simulink model "Complete_Sensorless_FOC_EKF_simulink_model"  (R2026a)
settings: Solver=ode23s  StopTime=inf  FixedStep=5e-5  MaxStep=1e-2
model workspace (MAT data in the model file):
  SL_ROS_VariableLengthArrays_MaxSizes.CommonInfo.ArrayTruncateAction = 'EmitWarning'
  SL_ROS_VariableLengthArrays_MaxSizes.MsgTypeMap = containers.Map
  SL_ROS_VariableLengthArrays_MaxSizes.MsgTypeMap.serialization.keys = {'std_msgs/Float64MultiArray'}
  SL_ROS_VariableLengthArrays_MaxSizes.MsgTypeMap.serialization.values{1}.PropertyName = 'data'
  SL_ROS_VariableLengthArrays_MaxSizes.MsgTypeMap.serialization.values{1}.DataType = 'double'
  SL_ROS_VariableLengthArrays_MaxSizes.MsgTypeMap.serialization.values{1}.MaxLength = 6
  SL_ROS_VariableLengthArrays_MaxSizes.MsgTypeMap.serialization.uniformity = 0
  SL_ROS_VariableLengthArrays_MaxSizes.MsgTypeMap.serialization.keyType = 'char'
  SL_ROS_VariableLengthArrays_MaxSizes.MsgTypeMap.serialization.valueType = 'any'
values from neighbouring files (symbols this model uses):
  id_ref = 0    [motor_params.m]
  J = 0.001    [motor_params.m]
  Kp_id = 37.7    [motor_params.m]
  Kp_iq = 65.97    [motor_params.m]
  lam = 0.175    [motor_params.m]
  Ld = 6e-3    (= 0.006)    [motor_params.m]
  Lq = 10.5e-3    (= 0.0105)    [motor_params.m]
  Ts = 50e-6    (= 5e-05)    [motor_params.m]
  V_dc = 48    [motor_params.m]
  V_lim = 27.7    [motor_params.m]
undefined symbols (not defined in the file or in its folder): data, data_SL_Info, DiscIntNeverNeededParam, dspblkCoreblockFVToolHelper, gcbh
libraries: nesl_utility x34, fl_lib x22, ee_lib x16, ros2lib x3
(part 1 of 2)
settings Model: Creator=vodna  LastModifiedBy=Hp
settings HardwareCC: UseEmbeddedCoderFeatures=off
settings RTWCC: SystemTargetFile=ert.tlc  HardwareBoard=Robot Operating System 2 (ROS 2)  TLCOptions="-aInlineSetEventsForThisBaseRateFcn=TLC_FALSE -aSuppressMultiTaskScheduler=TLC_FALSE  -aRateBasedStepFcn=0"  Toolchain=Colcon Tools  TargetLang=C++  Description=Embedded Coder
settings ERTTargetCC: ExtModeTransport=2.0  ExtModeAutomaticAllocSize=off  RootIOFormat=Structure reference  CodeInterfacePackaging=C++ class  SupportNonInlinedSFcns=on

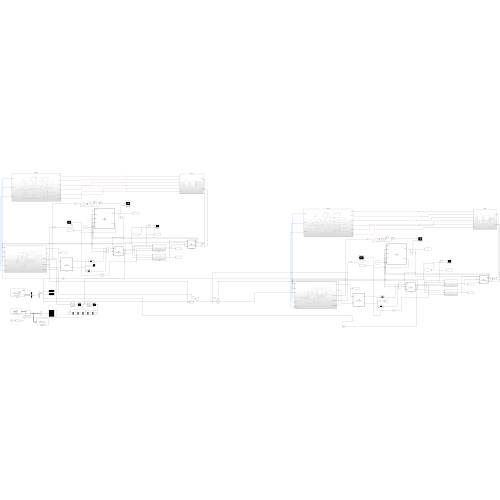
[thumbnail: Simulink's stored preview of the top-level diagram]
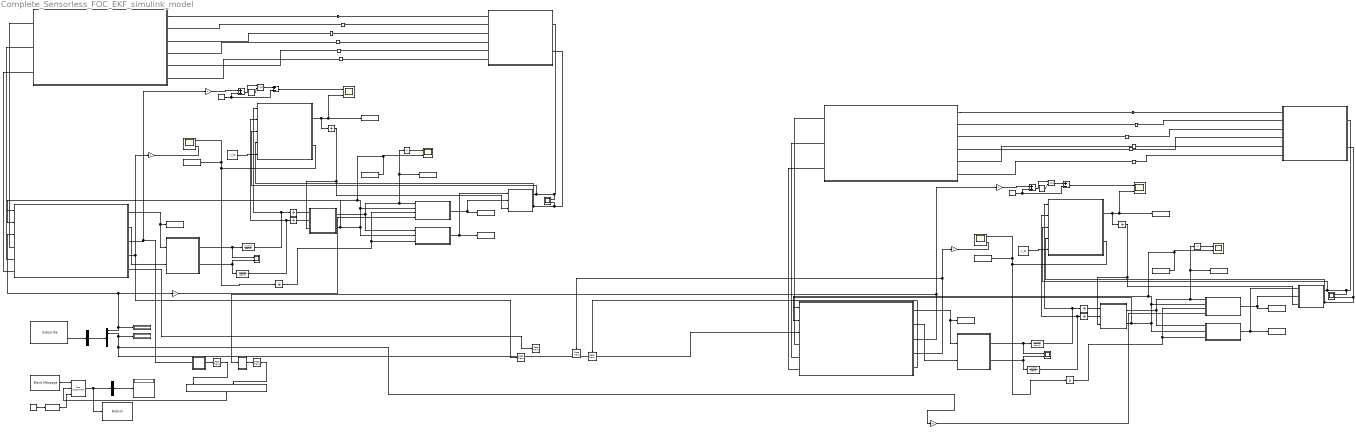
== system Complete_Sensorless_FOC_EKF_simulink_model ==
  Abs : Abs  SaturateOnIntegerOverflow=off
  Abs1 : Abs  SaturateOnIntegerOverflow=off
  Add : Sum
  Add1 : Sum  Inputs=+-
  Add2 : Sum
  Add3 : Sum  Inputs=+-
  Blank Message : ros2lib/Blank Message  messageClass=Message  entityType=std_msgs/Float64MultiArray  messageType=std_msgs/Float64MultiArray  SampleTime=-1
  Bus Assignment : BusAssignment  AssignedSignals=data,data_SL_Info.CurrentLength
  Bus Selector : BusSelector  OutputSignals=data
  Bus Selector1 : BusSelector  OutputSignals=data
  Constant : Constant  Value=pi
  Constant1 : Constant  Value=2*pi
  Constant10 : Constant  Value=pi
  Constant11 : Constant  Value=2*pi
  Constant12 : Constant  Value=V_dc
  Constant2 : Constant  Value=V_dc
  Constant9 : Constant  Value=6
  Data Type Conversion : DataTypeConversion  OutDataTypeStr=uint32  SaturateOnIntegerOverflow=off  RndMeth=Floor
  Demux : Demux  Outputs=6
  Discrete Filter{1..4} (4 alike) : DiscreteFilter  LoadFcn=dspblkCoreblockFVToolHelper(gcbh,'load');  Numerator=[0.00482434, 0.01929737, 0.02894606, 0.01929737, 0.00482434]  Denominator=[1.0, -2.36951300, 2.31398841, -1.05466541, 0.18737949]
      settings: CopyFcn=dspblkCoreblockFVToolHelper(gcbh,'copy');  DeleteFcn=dspblkCoreblockFVToolHelper(gcbh,'close');  ModelCloseFcn=dspblkCoreblockFVToolHelper(gcbh,'close');  PreSaveFcn=dspblkCoreblockFVToolHelper(gcbh,'presave');  PostSaveFcn=dspblkCoreblockFVToolHelper(gcbh,'postsave');  CloseFcn=dspblkCoreblockFVToolHelper(gcbh,'close');
  Display2 : Display
  Gain{,1..2,4} (4 alike) : Gain  Gain=4
  Gain3 : Gain  Gain=0.9524
  Gain5 : Gain  Gain=0.9524
  INVERTER : Subsystem
  INVERTER1 : Subsystem
  Id_PI : Subsystem
  Id_PI1 : Subsystem
  Inverse_park : MATLAB Function  TreatAsAtomicUnit=on
  Inverse_park1 : MATLAB Function  TreatAsAtomicUnit=on
  Iq_PI : Subsystem
  Iq_PI1 : Subsystem
  MATLAB Function1 : MATLAB Function  TreatAsAtomicUnit=on
  MATLAB Function2 : MATLAB Function  TreatAsAtomicUnit=on
  MOTOR : Subsystem
  MOTOR1 : Subsystem
  Mod : Math  Operator=mod
  Mod1 : Math  Operator=mod
  "Publish " : ros2lib/Publish  topicSource=Specify your own  topic=/leg/motor_feedback  messageType=std_msgs/Float64MultiArray  QOSHistory=Keep last  QOSDepth=10  QOSReliability=Reliable  QOSDurability=Volatile  QOSDeadline=Inf  QOSLifespan=Inf  QOSLiveliness=Automatic  QOSLeaseDuration=Inf  QOSAvoidROSNamespaceConventions=off
  Rate Transition{,1..5} (6 alike) : RateTransition
  SVPWM : Subsystem
  SVPWM1 : Subsystem
  Scope{,1..3} (4 alike) : Scope  NumInputPorts=2
      Scope settings: ActiveDisplayYMinimum=-7.5013972867973866  ActiveDisplayYMaximum=7.1966234186357241  DataLoggingVariableName=ScopeData2
      Scope1 settings: ActiveDisplayYMinimum=-7.5013972867973866  ActiveDisplayYMaximum=7.1966234186357241
      Scope2 settings: ActiveDisplayYMinimum=-37.09990453223314  ActiveDisplayYMaximum=28.788589033552036  DataLoggingVariableName=ScopeData6
      Scope3 settings: ActiveDisplayYMinimum=-37.09990453223314  ActiveDisplayYMaximum=28.788589033552036  DataLoggingVariableName=ScopeData13
  Scope_Angle : Scope  NumInputPorts=2
      settings: ActiveDisplayYMinimum=-0.32006576062717895  ActiveDisplayYMaximum=0.46001905422046974  DataLoggingVariableName=ScopeData5
  Scope_Angle1 : Scope  NumInputPorts=2
      settings: ActiveDisplayYMinimum=-17.181970691619213  ActiveDisplayYMaximum=15.500935335106382  DataLoggingVariableName=ScopeData12
  Scope_Speed1 : Scope  NumInputPorts=2
      settings: ActiveDisplayYMinimum=3.5802698086616154  ActiveDisplayYMaximum=53.8850630573057  DataLoggingVariableName=ScopeData14
  Scope_idq : Scope  NumInputPorts=2
      settings: ActiveDisplayYMinimum=-6.946558541995099  ActiveDisplayYMaximum=3.3320508183776947  DataLoggingVariableName=ScopeData8
  Scope_idq1 : Scope  NumInputPorts=2
      settings: ActiveDisplayYMinimum=-0.83754571636291986  ActiveDisplayYMaximum=0.92704548616719151  DataLoggingVariableName=ScopeData15
  Scope_theta : Scope  NumInputPorts=2
      settings: ActiveDisplayYMinimum=-1105.3552239828523  ActiveDisplayYMaximum=554.10895994113878  DataLoggingVariableName=ScopeData3
  Simulink-PS Converter{,1..11} (12 alike) : nesl_utility/Simulink-PS Converter  PhysicalDomain=network_engine_domain  SubClassName=ps_input  LeftPortType=input  RightPortType=output  PseudoPeriodic=off  Frequencies=[]  NoiseDistribution=none  NoiseParameters=[]  Unit=1  AffineConversion=off  FilteringAndDerivatives=provide  SimscapeFilterOrder=1  InputFilterTimeConstant=0.001  UdotUserProvided=0
  "Subscribe " : ros2lib/Subscribe  topicSource=Specify your own  topic=/leg/torque_cmd  messageType=std_msgs/Float64MultiArray  sampleTime=-1  QOSHistory=Keep last  QOSDepth=10  QOSReliability=Reliable  QOSDurability=Volatile  QOSDeadline=Inf  QOSLifespan=Inf  QOSLiveliness=Automatic  QOSLeaseDuration=Inf  QOSAvoidROSNamespaceConventions=off
  T_hip : Display
  T_knee : Display
  To Workspace : ToWorkspace  VariableName=speed_log  SampleTime=-1
  To Workspace1 : ToWorkspace  VariableName=rotor_angle  SampleTime=-1
  To Workspace10 : ToWorkspace  VariableName=vq_log1  SampleTime=-1
  To Workspace11 : ToWorkspace  VariableName=vd_log1  SampleTime=-1
  To Workspace12 : ToWorkspace  VariableName=iq_log1  SampleTime=-1
  To Workspace13 : ToWorkspace  VariableName=id_log1  SampleTime=-1
  To Workspace2 : ToWorkspace  VariableName=speed_log1  SampleTime=-1
  To Workspace3 : ToWorkspace  VariableName=rotor_angle1  SampleTime=-1
  To Workspace4 : ToWorkspace  VariableName=ia_log  SampleTime=-1
  To Workspace5 : ToWorkspace  VariableName=vq_log  SampleTime=-1
  To Workspace6 : ToWorkspace  VariableName=vd_log  SampleTime=-1
  To Workspace7 : ToWorkspace  VariableName=iq_log  SampleTime=-1
  To Workspace8 : ToWorkspace  VariableName=id_log  SampleTime=-1
  To Workspace9 : ToWorkspace  VariableName=ia_log1  SampleTime=-1
  Unit Delay{,1..2,4..7,9} (8 alike) : UnitDelay  SampleTime=Ts
  Vector Concatenate : Concatenate  NumInputs=6
  angle_wrap : Subsystem
  angle_wrap1 : Subsystem
  clarke : MATLAB Function  TreatAsAtomicUnit=on
  clarke1 : MATLAB Function  TreatAsAtomicUnit=on
  park : MATLAB Function  TreatAsAtomicUnit=on
  park1 : MATLAB Function  TreatAsAtomicUnit=on
  wires:
  clarke/2(i_beta) -> Discrete Filter2/1, Scope/2
  Abs/1 -> Scope_idq/1
  Unit Delay/1 -> park/1(i_alpha)
  Unit Delay1/1 -> park/2(i_beta)
  park/1(id) -> Abs/1, To Workspace8/1, Iq_PI/1(In1), Id_PI/1(In1)
  clarke/1(i_alpha) -> Scope/1, Discrete Filter1/1
  Inverse_park/1(v_alpha) -> MATLAB Function1/3(Valpha), Scope3/1, SVPWM/1(v_alpha)
  Inverse_park/2(v_beta) -> MATLAB Function1/4(Vbeta), Scope3/2, SVPWM/2(v_beta)
  Unit Delay2/1 -> Inverse_park/3(theta), park/3(theta)
  SVPWM/1(S1) -> Simulink-PS Converter/1
  SVPWM/5(S5) -> Simulink-PS Converter4/1
  SVPWM/4(S4) -> Simulink-PS Converter3/1
  SVPWM/6(S6) -> Simulink-PS Converter5/1
  SVPWM/3(S3) -> Simulink-PS Converter2/1
  SVPWM/2(S2) -> Simulink-PS Converter1/1
  Discrete Filter2/1 -> MATLAB Function1/2(Ibeta_filt), Unit Delay1/1
  Constant2/1 -> MATLAB Function1/5(Vdc)
  MATLAB Function1/1(theta_hat) -> Scope_Angle/2, To Workspace1/1, Unit Delay2/1
  Discrete Filter1/1 -> MATLAB Function1/1(Ialpha_filt), Unit Delay/1
  MATLAB Function1/2(omega_hat) -> Unit Delay4/1, To Workspace/1, Scope_theta/1
  MOTOR/1(ia) -> clarke/1(ia), To Workspace4/1
  MOTOR/2(ib) -> clarke/2(ib)
  Id_PI/1(Out1) -> To Workspace6/1, Inverse_park/1(vd)
  Iq_PI/1(Out1) -> To Workspace5/1, Inverse_park/2(vq)
  Demux/1 -> T_hip/1, Gain3/1, MOTOR/3(In1)  "T_hip"
  park/2(iq) -> Scope_idq/2, To Workspace7/1, MOTOR/1(iq), Iq_PI/2(In2), Id_PI/2(In2), MOTOR/2(id)
  Unit Delay4/1 -> Id_PI/3(In3), Iq_PI/3(In3)
  Gain/1 -> Scope_theta/2
  Constant/1 -> Add1/2, Add/2
  Add/1 -> Mod/1
  Constant1/1 -> Mod/2
  Mod/1 -> Add1/1
  Add1/1 -> Scope_Angle/1
  Gain1/1 -> Add/1
  Data Type Conversion/1 -> Bus Assignment/3
  MOTOR/3(theta_sensor) -> angle_wrap1/1(theta_hip), Gain1/1  "theta_hip"
  MOTOR/4(omega_sensor) -> Gain/1, Rate Transition2/1  "omega_hip"
  MOTOR1/4(omega_sensor) -> Rate Transition4/1, Gain2/1  "omega_knee"
  MOTOR/5(alpha_sensor) -> Rate Transition3/1  "alpha_hip"
  Constant9/1 -> Data Type Conversion/1
  MOTOR1/3(theta_sensor) -> Gain4/1, angle_wrap/1(theta_knee)  "theta_knee"
  Vector Concatenate/1 -> Bus Assignment/2
  Bus Selector1/1 -> Display2/1  "<data>"
  Blank Message/1 -> Bus Assignment/1
  Bus Assignment/1 -> "Publish "/1, Bus Selector1/1
  MOTOR1/5(alpha_sensor) -> Rate Transition5/1  "alpha_knee"
  Demux/2 -> MOTOR1/3(In1), Gain5/1, T_knee/1  "T_knee"
  "Subscribe "/2 -> Bus Selector/1
  Bus Selector/1 -> Demux/1  "<data>"
  Discrete Filter3/1 -> MATLAB Function2/1(Ialpha_filt), Unit Delay5/1
  Discrete Filter4/1 -> MATLAB Function2/2(Ibeta_filt), Unit Delay6/1
  Gain2/1 -> Scope_Speed1/2
  Add2/1 -> Mod1/1
  SVPWM1/6(S6) -> Simulink-PS Converter11/1
  Constant12/1 -> MATLAB Function2/5(Vdc)
  Unit Delay5/1 -> park1/1(i_alpha)
  MATLAB Function2/2(omega_hat) -> Unit Delay9/1, To Workspace2/1, Scope_Speed1/1
  Iq_PI1/1(Out1) -> To Workspace10/1, Inverse_park1/2(vq)
  clarke1/1(i_alpha) -> Scope1/1, Discrete Filter3/1
  SVPWM1/5(S5) -> Simulink-PS Converter10/1
  MOTOR1/1(ia) -> clarke1/1(ia), To Workspace9/1
  SVPWM1/4(S4) -> Simulink-PS Converter9/1
  park1/2(iq) -> Scope_idq1/2, To Workspace12/1, MOTOR1/1(iq), Iq_PI1/2(In2), Id_PI1/2(In2), MOTOR1/2(id)
  Mod1/1 -> Add3/1
  Inverse_park1/2(v_beta) -> MATLAB Function2/4(Vbeta), SVPWM1/2(v_beta), Scope2/2
  Constant11/1 -> Mod1/2
  clarke1/2(i_beta) -> Discrete Filter4/1, Scope1/2
  Inverse_park1/1(v_alpha) -> MATLAB Function2/3(Valpha), Scope2/1, SVPWM1/1(v_alpha)
  Id_PI1/1(Out1) -> To Workspace11/1, Inverse_park1/1(vd)
  Unit Delay9/1 -> Id_PI1/3(In3), Iq_PI1/3(In3)
  Constant10/1 -> Add3/2, Add2/2
  SVPWM1/3(S3) -> Simulink-PS Converter8/1
  MATLAB Function2/1(theta_hat) -> Scope_Angle1/2, To Workspace3/1, Unit Delay7/1
  MOTOR1/2(ib) -> clarke1/2(ib)
  Unit Delay7/1 -> Inverse_park1/3(theta), park1/3(theta)
  Unit Delay6/1 -> park1/2(i_beta)
  Gain4/1 -> Add2/1
  SVPWM1/1(S1) -> Simulink-PS Converter6/1
  Add3/1 -> Scope_Angle1/1
  park1/1(id) -> Abs1/1, To Workspace13/1, Iq_PI1/1(In1), Id_PI1/1(In1)
  Abs1/1 -> Scope_idq1/1
  Gain5/1 -> Iq_PI1/4(In4)
  SVPWM1/2(S2) -> Simulink-PS Converter7/1
  Gain3/1 -> Iq_PI/4(In4)
  Rate Transition/1 -> Vector Concatenate/1
  Rate Transition1/1 -> Vector Concatenate/4
  angle_wrap/1(Out1) -> Rate Transition1/1
  angle_wrap1/1(Out1) -> Rate Transition/1
  connections:
  INVERTER/LConn1 -- Simulink-PS Converter/RConn1
  Simulink-PS Converter1/RConn1 -- INVERTER/LConn2
  Simulink-PS Converter2/RConn1 -- INVERTER/LConn3
  Simulink-PS Converter3/RConn1 -- INVERTER/LConn4
  Simulink-PS Converter4/RConn1 -- INVERTER/LConn5
  Simulink-PS Converter5/RConn1 -- INVERTER/LConn6
  MOTOR/LConn2 -- INVERTER/RConn2
  MOTOR/LConn1 -- INVERTER/RConn1
  MOTOR/LConn3 -- INVERTER/RConn3
  INVERTER1/LConn1 -- Simulink-PS Converter6/RConn1
  Simulink-PS Converter7/RConn1 -- INVERTER1/LConn2
  MOTOR1/LConn3 -- INVERTER1/RConn3
  MOTOR1/LConn1 -- INVERTER1/RConn1
  Simulink-PS Converter8/RConn1 -- INVERTER1/LConn3
  Simulink-PS Converter9/RConn1 -- INVERTER1/LConn4
  Simulink-PS Converter10/RConn1 -- INVERTER1/LConn5
  MOTOR1/LConn2 -- INVERTER1/RConn2
  Simulink-PS Converter11/RConn1 -- INVERTER1/LConn6

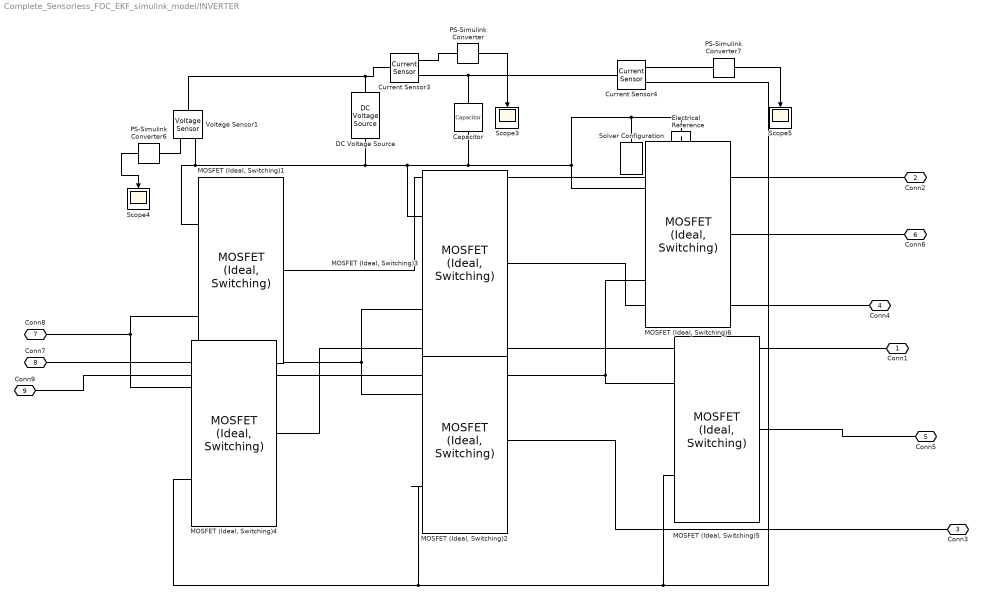
== system Complete_Sensorless_FOC_EKF_simulink_model/INVERTER ==
  Capacitor : fl_lib/Electrical/Electrical Elements/Capacitor  c=27e-6 F  r=1e-6 Ohm  g=0 1/Ohm  i_specify=off  i_priority=None  i=0 A  i_nominal_specify=off  i_nominal_value=1  i_nominal_unit=A  v_specify=off  v_priority=None  v=0 V  v_nominal_specify=off  v_nominal_value=1  v_nominal_unit=V  vc_specify=off  vc_priority=High  vc=0 V  vc_nominal_specify=off  vc_nominal_value=1  vc_nominal_unit=V
  Current Sensor3 : fl_lib/Electrical/Electrical Sensors/Current Sensor
  Current Sensor4 : fl_lib/Electrical/Electrical Sensors/Current Sensor
  DC Voltage Source : ee_lib/Additional Components/SPICE Sources/DC Voltage Source  DC=V_dc V
  Electrical Reference : fl_lib/Electrical/Electrical Elements/Electrical Reference
  MOSFET (Ideal, Switching){1..6} (6 alike) : ee_lib/Semiconductors & Converters/MOSFET (Ideal, Switching)  port_option=ee.enum.controlport.ps  Rds=0.0175 Ohm  Goff=1e-6 1/Ohm  Vth=0.5 V  diode_param=ee.enum.semiconductors.protectionDiode.nodynamics  diode_Vf=0.9 V  diode_Ron=0.001 Ohm  diode_Goff=1e-5 1/Ohm  diode_C=50e-9 F  diode_iRM=-235 A  diode_iF=300 A  diode_idot=-50 A/us  diode_trr_param=ee.enum.converters.diodeReverseParam.trr_factor  diode_trr_factor=3  diode_trr=15 us  diode_Qrr=1500 s*uA  ids_specify=off  ids_priority=None  ids=0 A  ids_nominal_specify=off  ids_nominal_value=1  ids_nominal_unit=A  vds_specify=off  vds_priority=None  vds=0 V  vds_nominal_specify=off  vds_nominal_value=1  vds_nominal_unit=V  vgs_specify=off  vgs_priority=None  vgs=0 V  vgs_nominal_specify=off  vgs_nominal_value=1  vgs_nominal_unit=V  thermal_loss_option=ee.enum.converters.thermalLossOption.constantvalues  Von_data=[0, 1.8, 3.2, 6, 10, 16; 0, 2, 5.5, 9.5, 15, 25] V  Tj=[298.15, 448.15] K  Iout_data=[0, 20, 40, 60, 80, 100] A  tabulateWithVds=false  Eon_data=[0, 55.04, 124.57, 235.53, 362.12; 0, 71.25, 161.25, 304.88, 468.75] * 1e-6 J  Eoff_data=[0, 18, 30, 56.1, 76.5; 0, 22.5, 37.5, 70.13, 95.63] * 1e-6 J  Eon_data_3D=[zeros(2, 5, 3)] J  Eoff_data_3D=[zeros(2, 5, 3)] J  Tj_loss=[298.15, 448.15] K  Iout_data_loss=[0, 10, 20, 30, 40] A  Vds_loss=[0, 150, 300] V  Eon_scalar=22.86e-3 J  Eoff_scalar=17.14e-3 J  Voff=300 V  Iout_scalar=600 A  useCurrentFromPreviousCycle=false  useVoltageFromPreviousCycle=false  diodeModelType=ee.enum.converters.diodeModelType.pwl  diodeTableType=ee.enum.diode.tableType.IfMat  diode_ReverseIVType=ee.enum.diode.diodeReverseIV.constant  diode_IfMat=[.07, .12, .19, 1.75, 4.24, 7.32, 11.2; .16, .3, .72, 2.14, 4.02, 6.35, 9.12] A  diode_VfMat=[.9, 1.15, 1.25, 1.5, 1.75, 2.17, 2.6, 2.85; .58, .68, .75, 1.1, 1.38, 1.77, 2.27, 2.7] V  diode_TjVec=[25, 125] degC  diode_VfVec=[.5, .7, .9, 1.3, 1.7, 2.1, 2.5] V  diode_IfVec=[.1, .2, .5, 1, 2, 4, 7, 10] A  diode_IrMat=[1e-06, 2e-06, 5e-06, 1e-05, 2.5e-05, 5e-05, .0001; 2e-06, 5e-06, 1e-05, 4e-05, 8e-05, .0002, .0005] A  diode_VrMat=[10, 100, 200, 250, 300, 325, 350; 10, 70, 160, 220, 270, 300, 320] V  diode_VrVec=[10, 20, 40, 50, 70, 80, 100] V  diode_IrVec=[1e-06, 2e-06, 5e-06, 1e-05, 2e-05, 5e-05, .0001] A  diode_Vr=-600 V  diode_Ls=150 nH  diode_Erec=0.03 J  diode_rec_loss_model=ee.enum.diode.reverseRecoveryModelTabulateUpTo3D.fixed  diode_ErecVal=0 J  diode_scaleWithIandV=true  diode_ErecMat=zeros(2, 3) J  diodeErecMat3D=zeros(2, 3, 2) J  diode_TjrecVec=[298.15, 398.15] K  diode_IfrecVec=[.1, 1, 10] A  diodeVrecVec=[0, 100] V  diode_IrecVal=10 A  diode_VrecVal=10 V  diode_tFilter=1 / 1000 / 100 s  separateThermalPortForDiode=false  thermal_network_parameterization=ee.enum.thermalNetworkTopology.external  Rth=[.03, .2] K/W  Rth_Cauer=[.03, .1, .2] K/W  Rth_Foster=[.08, .14, .22, .16] K/W  thermal_mass_parameterization=ee.enum.thermalNetwork.timeconstant  thermal_mass=[3, 25] J/K  thermal_mass_Cauer=[3, 10, 25] J/K  thermal_mass_Foster=[.001, .005, .05, .5] J/K  thermal_time_constant=[.1, 5] s  thermal_time_constant_Cauer=[.1, 1, 5] s  thermal_time_constant_Foster=[7e-05, .0007, .01, .08] s  thermal_mass_initial_temperatures=[25, 25] degC  thermal_mass_initial_temperatures_Cauer=[25, 25, 25] degC  junction_thermal_mass=0.1 J/K  Tvec_initial_Foster=[25, 25, 25, 25] degC  RthDiode=[.03, .2] K/W  RthCauerDiode=[.03, .1, .2] K/W  RthFosterDiode=[.03, .2] K/W  thermalMassDiode=[3, 25] J/K  thermalMassCauerDiode=[3, 10, 25] J/K  thermalMassFosterDiode=[33, 50] J/K  thermalTauDiode=[.1, 5] s  thermalTauCauerDiode=[.1, 1, 5] s  thermalTauFosterDiode=[1, 10] s  thermalMassInitTempDiode=[25, 25] degC  thermalMassInitTempCauerDiode=[25, 25, 25] degC  junctionthermalMassDiode=0.1 J/K  TVecInitialFosterDiode=[25, 25, 25, 25] degC  no_thermal_network=ee.enum.enable.no  mosfet_junction_temperature_specify=off  mosfet_junction_temperature_priority=None  mosfet_junction_temperature=25 degC  mosfet_junction_temperature_nominal_specify=off  mosfet_junction_temperature_nominal_value=1  mosfet_junction_temperature_nominal_unit=degC  diode_junction_temperature_specify=off  diode_junction_temperature_priority=None  diode_junction_temperature=25 degC  diode_junction_temperature_nominal_specify=off  diode_junction_temperature_nominal_value=1  diode_junction_temperature_nominal_unit=degC  Qj_specify=off  Qj_priority=None  Qj=0 W  Qj_nominal_specify=off  Qj_nominal_value=1  Qj_nominal_unit=W  accumulatedSwitchingLosses_specify=off  accumulatedSwitchingLosses_priority=None  accumulatedSwitchingLosses=0 J
  PS-Simulink Converter : nesl_utility/PS-Simulink Converter  PhysicalDomain=network_engine_domain  SubClassName=ps_output  LeftPortType=input  RightPortType=output  PseudoPeriodic=off  Frequencies=[]  VectorFormat=inherit  Unit=inherit  AffineConversion=off
  PS-Simulink Converter6 : nesl_utility/PS-Simulink Converter  PhysicalDomain=network_engine_domain  SubClassName=ps_output  LeftPortType=input  RightPortType=output  PseudoPeriodic=off  Frequencies=[]  VectorFormat=inherit  Unit=inherit  AffineConversion=off
  PS-Simulink Converter7 : nesl_utility/PS-Simulink Converter  PhysicalDomain=network_engine_domain  SubClassName=ps_output  LeftPortType=input  RightPortType=output  PseudoPeriodic=off  Frequencies=[]  VectorFormat=inherit  Unit=inherit  AffineConversion=off
  Scope3 : Scope
      settings: ActiveDisplayYMinimum=-6.000118872312692E+6  ActiveDisplayYMaximum=5.4000013209794745E+7  DataLoggingVariableName=ScopeData4
  Scope4 : Scope
      settings: ActiveDisplayYMinimum=38  ActiveDisplayYMaximum=58  DataLoggingVariableName=ScopeData10
  Scope5 : Scope
      settings: ActiveDisplayYMinimum=-1.3368858719998875  ActiveDisplayYMaximum=5.5423081555367419  DataLoggingVariableName=ScopeData11
  Solver Configuration : nesl_utility/Solver Configuration  PhysicalDomain=network_engine_domain  SubClassName=solver  LeftPortType=input  RightPortType=generic  Tones=[]  Harmonics=[]  SimulateNoise=off  Profile=off  UseLocalSampling=off  EnableSwitchedLinearOptims=on  FrequencyDomain=off  UseCCode=off  RelTol=0.001  AbsTol=0.001  MinStep=1e-09  ToWorkspace=off  RevertToSquareIcSolve=off  NumHomotopyIterations=100  PhasorMode=off  PhasorModeNumHarmonics=1  ConsistencySolver=NEWTON_XTOL_AFTER_FTOL  CanonicalOrdering=CANONICAL  OptimizeIntermediates=OPTIMIZED  IndexReductionMethod=DerivativeReplacement  DoDC=off  ResidualTolerance=1e-09  ConsistencyTolSource=GLOBAL  ConsistencyAbsTol=0.001  ConsistencyRelTol=0.001  ConsistencyTolFactor=0.001  UseLocalSolver=off  LocalSolverChoice=NE_BACKWARD_EULER_ADVANCER  ResolveIndetEquations=on  FunctionEvalNumThread=1  LocalSolverSampleTime=0.001  DoFixedCost=off  MaxNonlinIter=3  MaxModeIter=2  ComputeImpulses=off  ImpulseIterations=2  LinearAlgebra=auto  LinearAlgebraNumThread=0  EquationFormulation=NE_TIME_EF  DelaysMemoryBudget=1024  AutomaticFiltering=on  FilteringTimeConstant=0.001  PartitionStorageMethod=AS_NEEDED  PartitionMemoryBudget=1024  PartitionMethod=ROBUST  MultibodyUseLocalSolver=off  MultibodyLocalSolverChoice=ODE1  MultibodyLocalSolverSampleTime=0.001
  Voltage Sensor1 : fl_lib/Electrical/Electrical Sensors/Voltage Sensor
  Conn1 : PMIOPort  Side=Left
  Conn2 : PMIOPort  Port=2  Side=Left
  Conn3 : PMIOPort  Port=3  Side=Left
  Conn4 : PMIOPort  Port=4  Side=Left
  Conn5 : PMIOPort  Port=5  Side=Left
  Conn6 : PMIOPort  Port=6  Side=Left
  Conn8 : PMIOPort  Port=7  Side=Right
  Conn7 : PMIOPort  Port=8  Side=Right
  Conn9 : PMIOPort  Port=9  Side=Right
  wires:
  PS-Simulink Converter6/1 -> Scope4/1
  PS-Simulink Converter/1 -> Scope3/1
  PS-Simulink Converter7/1 -> Scope5/1
  connections:
  "MOSFET (Ideal, Switching)3"/RConn2 -- "MOSFET (Ideal, Switching)1"/RConn2 -- Voltage Sensor1/RConn2 -- DC Voltage Source/RConn1 -- Electrical Reference/LConn1 -- Solver Configuration/RConn1 -- "MOSFET (Ideal, Switching)6"/RConn2 -- Capacitor/RConn1
  Conn4/RConn1 -- "MOSFET (Ideal, Switching)3"/LConn1
  Conn2/RConn1 -- "MOSFET (Ideal, Switching)1"/LConn1
  "MOSFET (Ideal, Switching)6"/RConn1 -- "MOSFET (Ideal, Switching)5"/RConn2 -- Conn9/RConn1
  DC Voltage Source/LConn1 -- Voltage Sensor1/LConn1 -- Current Sensor3/LConn1
  Current Sensor3/RConn2 -- Current Sensor4/LConn1 -- Capacitor/LConn1
  Conn8/RConn1 -- "MOSFET (Ideal, Switching)4"/RConn2 -- "MOSFET (Ideal, Switching)1"/RConn1
  PS-Simulink Converter/LConn1 -- Current Sensor3/RConn1
  PS-Simulink Converter6/LConn1 -- Voltage Sensor1/RConn1
  "MOSFET (Ideal, Switching)3"/RConn1 -- Conn7/RConn1 -- "MOSFET (Ideal, Switching)2"/RConn2
  PS-Simulink Converter7/LConn1 -- Current Sensor4/RConn1
  "MOSFET (Ideal, Switching)4"/RConn1 -- "MOSFET (Ideal, Switching)5"/RConn1 -- Current Sensor4/RConn2 -- "MOSFET (Ideal, Switching)2"/RConn1
  "MOSFET (Ideal, Switching)4"/LConn1 -- Conn1/RConn1
  Conn3/RConn1 -- "MOSFET (Ideal, Switching)2"/LConn1
  Conn5/RConn1 -- "MOSFET (Ideal, Switching)5"/LConn1
  Conn6/RConn1 -- "MOSFET (Ideal, Switching)6"/LConn1

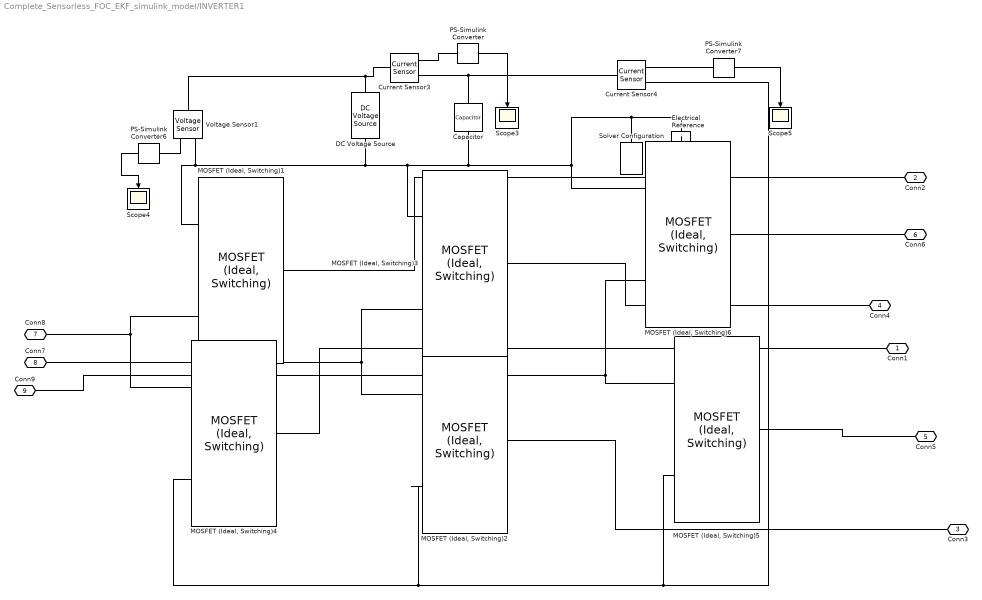
== system Complete_Sensorless_FOC_EKF_simulink_model/INVERTER1 ==
  Capacitor : fl_lib/Electrical/Electrical Elements/Capacitor  c=27e-6 F  r=1e-6 Ohm  g=0 1/Ohm  i_specify=off  i_priority=None  i=0 A  i_nominal_specify=off  i_nominal_value=1  i_nominal_unit=A  v_specify=off  v_priority=None  v=0 V  v_nominal_specify=off  v_nominal_value=1  v_nominal_unit=V  vc_specify=off  vc_priority=High  vc=0 V  vc_nominal_specify=off  vc_nominal_value=1  vc_nominal_unit=V
  Current Sensor3 : fl_lib/Electrical/Electrical Sensors/Current Sensor
  Current Sensor4 : fl_lib/Electrical/Electrical Sensors/Current Sensor
  DC Voltage Source : ee_lib/Additional Components/SPICE Sources/DC Voltage Source  DC=V_dc V
  Electrical Reference : fl_lib/Electrical/Electrical Elements/Electrical Reference
  MOSFET (Ideal, Switching){1..6} (6 alike) : ee_lib/Semiconductors & Converters/MOSFET (Ideal, Switching)  port_option=ee.enum.controlport.ps  Rds=0.0175 Ohm  Goff=1e-6 1/Ohm  Vth=0.5 V  diode_param=ee.enum.semiconductors.protectionDiode.nodynamics  diode_Vf=0.9 V  diode_Ron=0.001 Ohm  diode_Goff=1e-5 1/Ohm  diode_C=50e-9 F  diode_iRM=-235 A  diode_iF=300 A  diode_idot=-50 A/us  diode_trr_param=ee.enum.converters.diodeReverseParam.trr_factor  diode_trr_factor=3  diode_trr=15 us  diode_Qrr=1500 s*uA  ids_specify=off  ids_priority=None  ids=0 A  ids_nominal_specify=off  ids_nominal_value=1  ids_nominal_unit=A  vds_specify=off  vds_priority=None  vds=0 V  vds_nominal_specify=off  vds_nominal_value=1  vds_nominal_unit=V  vgs_specify=off  vgs_priority=None  vgs=0 V  vgs_nominal_specify=off  vgs_nominal_value=1  vgs_nominal_unit=V  thermal_loss_option=ee.enum.converters.thermalLossOption.constantvalues  Von_data=[0, 1.8, 3.2, 6, 10, 16; 0, 2, 5.5, 9.5, 15, 25] V  Tj=[298.15, 448.15] K  Iout_data=[0, 20, 40, 60, 80, 100] A  tabulateWithVds=false  Eon_data=[0, 55.04, 124.57, 235.53, 362.12; 0, 71.25, 161.25, 304.88, 468.75] * 1e-6 J  Eoff_data=[0, 18, 30, 56.1, 76.5; 0, 22.5, 37.5, 70.13, 95.63] * 1e-6 J  Eon_data_3D=[zeros(2, 5, 3)] J  Eoff_data_3D=[zeros(2, 5, 3)] J  Tj_loss=[298.15, 448.15] K  Iout_data_loss=[0, 10, 20, 30, 40] A  Vds_loss=[0, 150, 300] V  Eon_scalar=22.86e-3 J  Eoff_scalar=17.14e-3 J  Voff=300 V  Iout_scalar=600 A  useCurrentFromPreviousCycle=false  useVoltageFromPreviousCycle=false  diodeModelType=ee.enum.converters.diodeModelType.pwl  diodeTableType=ee.enum.diode.tableType.IfMat  diode_ReverseIVType=ee.enum.diode.diodeReverseIV.constant  diode_IfMat=[.07, .12, .19, 1.75, 4.24, 7.32, 11.2; .16, .3, .72, 2.14, 4.02, 6.35, 9.12] A  diode_VfMat=[.9, 1.15, 1.25, 1.5, 1.75, 2.17, 2.6, 2.85; .58, .68, .75, 1.1, 1.38, 1.77, 2.27, 2.7] V  diode_TjVec=[25, 125] degC  diode_VfVec=[.5, .7, .9, 1.3, 1.7, 2.1, 2.5] V  diode_IfVec=[.1, .2, .5, 1, 2, 4, 7, 10] A  diode_IrMat=[1e-06, 2e-06, 5e-06, 1e-05, 2.5e-05, 5e-05, .0001; 2e-06, 5e-06, 1e-05, 4e-05, 8e-05, .0002, .0005] A  diode_VrMat=[10, 100, 200, 250, 300, 325, 350; 10, 70, 160, 220, 270, 300, 320] V  diode_VrVec=[10, 20, 40, 50, 70, 80, 100] V  diode_IrVec=[1e-06, 2e-06, 5e-06, 1e-05, 2e-05, 5e-05, .0001] A  diode_Vr=-600 V  diode_Ls=150 nH  diode_Erec=0.03 J  diode_rec_loss_model=ee.enum.diode.reverseRecoveryModelTabulateUpTo3D.fixed  diode_ErecVal=0 J  diode_scaleWithIandV=true  diode_ErecMat=zeros(2, 3) J  diodeErecMat3D=zeros(2, 3, 2) J  diode_TjrecVec=[298.15, 398.15] K  diode_IfrecVec=[.1, 1, 10] A  diodeVrecVec=[0, 100] V  diode_IrecVal=10 A  diode_VrecVal=10 V  diode_tFilter=1 / 1000 / 100 s  separateThermalPortForDiode=false  thermal_network_parameterization=ee.enum.thermalNetworkTopology.external  Rth=[.03, .2] K/W  Rth_Cauer=[.03, .1, .2] K/W  Rth_Foster=[.08, .14, .22, .16] K/W  thermal_mass_parameterization=ee.enum.thermalNetwork.timeconstant  thermal_mass=[3, 25] J/K  thermal_mass_Cauer=[3, 10, 25] J/K  thermal_mass_Foster=[.001, .005, .05, .5] J/K  thermal_time_constant=[.1, 5] s  thermal_time_constant_Cauer=[.1, 1, 5] s  thermal_time_constant_Foster=[7e-05, .0007, .01, .08] s  thermal_mass_initial_temperatures=[25, 25] degC  thermal_mass_initial_temperatures_Cauer=[25, 25, 25] degC  junction_thermal_mass=0.1 J/K  Tvec_initial_Foster=[25, 25, 25, 25] degC  RthDiode=[.03, .2] K/W  RthCauerDiode=[.03, .1, .2] K/W  RthFosterDiode=[.03, .2] K/W  thermalMassDiode=[3, 25] J/K  thermalMassCauerDiode=[3, 10, 25] J/K  thermalMassFosterDiode=[33, 50] J/K  thermalTauDiode=[.1, 5] s  thermalTauCauerDiode=[.1, 1, 5] s  thermalTauFosterDiode=[1, 10] s  thermalMassInitTempDiode=[25, 25] degC  thermalMassInitTempCauerDiode=[25, 25, 25] degC  junctionthermalMassDiode=0.1 J/K  TVecInitialFosterDiode=[25, 25, 25, 25] degC  no_thermal_network=ee.enum.enable.no  mosfet_junction_temperature_specify=off  mosfet_junction_temperature_priority=None  mosfet_junction_temperature=25 degC  mosfet_junction_temperature_nominal_specify=off  mosfet_junction_temperature_nominal_value=1  mosfet_junction_temperature_nominal_unit=degC  diode_junction_temperature_specify=off  diode_junction_temperature_priority=None  diode_junction_temperature=25 degC  diode_junction_temperature_nominal_specify=off  diode_junction_temperature_nominal_value=1  diode_junction_temperature_nominal_unit=degC  Qj_specify=off  Qj_priority=None  Qj=0 W  Qj_nominal_specify=off  Qj_nominal_value=1  Qj_nominal_unit=W  accumulatedSwitchingLosses_specify=off  accumulatedSwitchingLosses_priority=None  accumulatedSwitchingLosses=0 J
  PS-Simulink Converter : nesl_utility/PS-Simulink Converter  PhysicalDomain=network_engine_domain  SubClassName=ps_output  LeftPortType=input  RightPortType=output  PseudoPeriodic=off  Frequencies=[]  VectorFormat=inherit  Unit=inherit  AffineConversion=off
  PS-Simulink Converter6 : nesl_utility/PS-Simulink Converter  PhysicalDomain=network_engine_domain  SubClassName=ps_output  LeftPortType=input  RightPortType=output  PseudoPeriodic=off  Frequencies=[]  VectorFormat=inherit  Unit=inherit  AffineConversion=off
  PS-Simulink Converter7 : nesl_utility/PS-Simulink Converter  PhysicalDomain=network_engine_domain  SubClassName=ps_output  LeftPortType=input  RightPortType=output  PseudoPeriodic=off  Frequencies=[]  VectorFormat=inherit  Unit=inherit  AffineConversion=off
  Scope3 : Scope
      settings: ActiveDisplayYMinimum=-6.000118872312692E+6  ActiveDisplayYMaximum=5.4000013209794745E+7  DataLoggingVariableName=ScopeData4
  Scope4 : Scope
      settings: ActiveDisplayYMinimum=38  ActiveDisplayYMaximum=58  DataLoggingVariableName=ScopeData10
  Scope5 : Scope
      settings: ActiveDisplayYMinimum=-1.3368858719998875  ActiveDisplayYMaximum=5.5423081555367419  DataLoggingVariableName=ScopeData11
  Solver Configuration : nesl_utility/Solver Configuration  PhysicalDomain=network_engine_domain  SubClassName=solver  LeftPortType=input  RightPortType=generic  Tones=[]  Harmonics=[]  SimulateNoise=off  Profile=off  UseLocalSampling=off  EnableSwitchedLinearOptims=on  FrequencyDomain=off  UseCCode=off  RelTol=0.001  AbsTol=0.001  MinStep=1e-09  ToWorkspace=off  RevertToSquareIcSolve=off  NumHomotopyIterations=100  PhasorMode=off  PhasorModeNumHarmonics=1  ConsistencySolver=NEWTON_XTOL_AFTER_FTOL  CanonicalOrdering=CANONICAL  OptimizeIntermediates=OPTIMIZED  IndexReductionMethod=DerivativeReplacement  DoDC=off  ResidualTolerance=1e-09  ConsistencyTolSource=GLOBAL  ConsistencyAbsTol=0.001  ConsistencyRelTol=0.001  ConsistencyTolFactor=0.001  UseLocalSolver=off  LocalSolverChoice=NE_BACKWARD_EULER_ADVANCER  ResolveIndetEquations=on  FunctionEvalNumThread=1  LocalSolverSampleTime=0.001  DoFixedCost=off  MaxNonlinIter=3  MaxModeIter=2  ComputeImpulses=off  ImpulseIterations=2  LinearAlgebra=auto  LinearAlgebraNumThread=0  EquationFormulation=NE_TIME_EF  DelaysMemoryBudget=1024  AutomaticFiltering=on  FilteringTimeConstant=0.001  PartitionStorageMethod=AS_NEEDED  PartitionMemoryBudget=1024  PartitionMethod=ROBUST  MultibodyUseLocalSolver=off  MultibodyLocalSolverChoice=ODE1  MultibodyLocalSolverSampleTime=0.001
  Voltage Sensor1 : fl_lib/Electrical/Electrical Sensors/Voltage Sensor
  Conn1 : PMIOPort  Side=Left
  Conn2 : PMIOPort  Port=2  Side=Left
  Conn3 : PMIOPort  Port=3  Side=Left
  Conn4 : PMIOPort  Port=4  Side=Left
  Conn5 : PMIOPort  Port=5  Side=Left
  Conn6 : PMIOPort  Port=6  Side=Left
  Conn8 : PMIOPort  Port=7  Side=Right
  Conn7 : PMIOPort  Port=8  Side=Right
  Conn9 : PMIOPort  Port=9  Side=Right
  wires:
  PS-Simulink Converter6/1 -> Scope4/1
  PS-Simulink Converter/1 -> Scope3/1
  PS-Simulink Converter7/1 -> Scope5/1
  connections:
  "MOSFET (Ideal, Switching)1"/RConn2 -- Voltage Sensor1/RConn2 -- DC Voltage Source/RConn1 -- "MOSFET (Ideal, Switching)3"/RConn2 -- Electrical Reference/LConn1 -- Solver Configuration/RConn1 -- "MOSFET (Ideal, Switching)6"/RConn2 -- Capacitor/RConn1
  Conn4/RConn1 -- "MOSFET (Ideal, Switching)3"/LConn1
  Conn2/RConn1 -- "MOSFET (Ideal, Switching)1"/LConn1
  "MOSFET (Ideal, Switching)6"/RConn1 -- "MOSFET (Ideal, Switching)5"/RConn2 -- Conn9/RConn1
  DC Voltage Source/LConn1 -- Voltage Sensor1/LConn1 -- Current Sensor3/LConn1
  Current Sensor3/RConn2 -- Current Sensor4/LConn1 -- Capacitor/LConn1
  Conn8/RConn1 -- "MOSFET (Ideal, Switching)4"/RConn2 -- "MOSFET (Ideal, Switching)1"/RConn1
  PS-Simulink Converter/LConn1 -- Current Sensor3/RConn1
  PS-Simulink Converter6/LConn1 -- Voltage Sensor1/RConn1
  "MOSFET (Ideal, Switching)3"/RConn1 -- Conn7/RConn1 -- "MOSFET (Ideal, Switching)2"/RConn2
  PS-Simulink Converter7/LConn1 -- Current Sensor4/RConn1
  "MOSFET (Ideal, Switching)5"/RConn1 -- Current Sensor4/RConn2 -- "MOSFET (Ideal, Switching)4"/RConn1 -- "MOSFET (Ideal, Switching)2"/RConn1
  "MOSFET (Ideal, Switching)4"/LConn1 -- Conn1/RConn1
  Conn3/RConn1 -- "MOSFET (Ideal, Switching)2"/LConn1
  Conn5/RConn1 -- "MOSFET (Ideal, Switching)5"/LConn1
  Conn6/RConn1 -- "MOSFET (Ideal, Switching)6"/LConn1

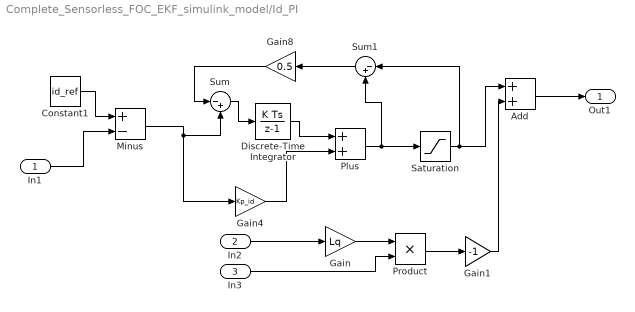
== system Complete_Sensorless_FOC_EKF_simulink_model/Id_PI ==
  In1 : Inport
  In2 : Inport  Port=2
  In3 : Inport  Port=3
  Add : Sum
  Constant1 : Constant  Value=id_ref  SampleTime=Ts
  Discrete-Time Integrator : DiscreteIntegrator  gainval=Kp_id  SampleTime=Ts  LimitOutput=on  UpperSaturationLimit=V_lim  LowerSaturationLimit=-V_lim  ICPrevOutput=DiscIntNeverNeededParam  ICPrevScaledInput=DiscIntNeverNeededParam
  Gain : Gain  Gain=Lq
  Gain1 : Gain  Gain=-1
  Gain4 : Gain  Gain=Kp_id
  Gain8 : Gain  Gain=0.5
  Minus : Sum  Inputs=+-
  Plus : Sum
  Product : Product
  Saturation : Saturate  UpperLimit=V_lim  LowerLimit=-V_lim
  Sum : Sum  Inputs=|-+
  Sum1 : Sum  Inputs=|-+
  Out1 : Outport
  wires:
  Constant1/1 -> Minus/1
  Saturation/1 -> Add/1, Sum1/1
  Gain8/1 -> Sum/1
  Sum1/1 -> Gain8/1
  Product/1 -> Gain1/1
  Gain4/1 -> Plus/2
  Gain/1 -> Product/1
  Gain1/1 -> Add/2
  Plus/1 -> Sum1/2, Saturation/1
  Minus/1 -> Sum/2, Gain4/1
  Discrete-Time Integrator/1 -> Plus/1
  In3/1 -> Product/2
  Sum/1 -> Discrete-Time Integrator/1
  In1/1 -> Minus/2
  Add/1 -> Out1/1
  In2/1 -> Gain/1

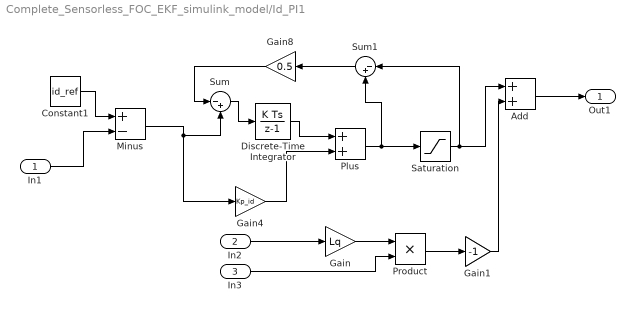
== system Complete_Sensorless_FOC_EKF_simulink_model/Id_PI1 ==
  In1 : Inport
  In2 : Inport  Port=2
  In3 : Inport  Port=3
  Add : Sum
  Constant1 : Constant  Value=id_ref  SampleTime=Ts
  Discrete-Time Integrator : DiscreteIntegrator  gainval=Kp_id  SampleTime=Ts  LimitOutput=on  UpperSaturationLimit=V_lim  LowerSaturationLimit=-V_lim  ICPrevOutput=DiscIntNeverNeededParam  ICPrevScaledInput=DiscIntNeverNeededParam
  Gain : Gain  Gain=Lq
  Gain1 : Gain  Gain=-1
  Gain4 : Gain  Gain=Kp_id
  Gain8 : Gain  Gain=0.5
  Minus : Sum  Inputs=+-
  Plus : Sum
  Product : Product
  Saturation : Saturate  UpperLimit=V_lim  LowerLimit=-V_lim
  Sum : Sum  Inputs=|-+
  Sum1 : Sum  Inputs=|-+
  Out1 : Outport
  wires:
  Constant1/1 -> Minus/1
  Saturation/1 -> Add/1, Sum1/1
  Gain8/1 -> Sum/1
  Sum1/1 -> Gain8/1
  Product/1 -> Gain1/1
  Gain4/1 -> Plus/2
  Gain/1 -> Product/1
  Gain1/1 -> Add/2
  Plus/1 -> Sum1/2, Saturation/1
  Minus/1 -> Sum/2, Gain4/1
  Discrete-Time Integrator/1 -> Plus/1
  In3/1 -> Product/2
  Sum/1 -> Discrete-Time Integrator/1
  In1/1 -> Minus/2
  Add/1 -> Out1/1
  In2/1 -> Gain/1

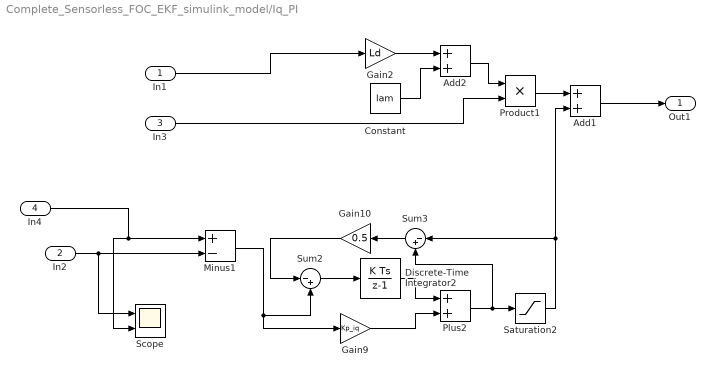
== system Complete_Sensorless_FOC_EKF_simulink_model/Iq_PI ==
  In1 : Inport
  In2 : Inport  Port=2
  In3 : Inport  Port=3
  In4 : Inport  Port=4
  Add1 : Sum
  Add2 : Sum
  Constant : Constant  Value=lam  VectorParams1D=off
  Discrete-Time Integrator2 : DiscreteIntegrator  gainval=Kp_iq  SampleTime=Ts  LimitOutput=on  UpperSaturationLimit=V_lim  LowerSaturationLimit=-V_lim  ICPrevOutput=DiscIntNeverNeededParam  ICPrevScaledInput=DiscIntNeverNeededParam
  Gain10 : Gain  Gain=0.5
  Gain2 : Gain  Gain=Ld
  Gain9 : Gain  Gain=Kp_iq
  Minus1 : Sum  Inputs=+-
  Plus2 : Sum
  Product1 : Product
  Saturation2 : Saturate  UpperLimit=V_lim  LowerLimit=-V_lim
  Scope : Scope  NumInputPorts=2
      settings: ActiveDisplayYMinimum=-4.4913250364505462E+6  ActiveDisplayYMaximum=4.180130070139687E+6  DataLoggingVariableName=ScopeData16
  Sum2 : Sum  Inputs=|-+
  Sum3 : Sum  Inputs=|-+
  Out1 : Outport
  wires:
  Minus1/1 -> Sum2/2, Gain9/1
  Saturation2/1 -> Sum3/1, Add1/2
  Add2/1 -> Product1/1
  Gain2/1 -> Add2/1
  Constant/1 -> Add2/2
  In3/1 -> Product1/2
  Gain9/1 -> Plus2/2
  Discrete-Time Integrator2/1 -> Plus2/1
  Plus2/1 -> Sum3/2, Saturation2/1
  Gain10/1 -> Sum2/1
  In1/1 -> Gain2/1
  Sum2/1 -> Discrete-Time Integrator2/1
  Product1/1 -> Add1/1
  Sum3/1 -> Gain10/1
  Add1/1 -> Out1/1
  In2/1 -> Scope/1, Minus1/2
  In4/1 -> Scope/2, Minus1/1

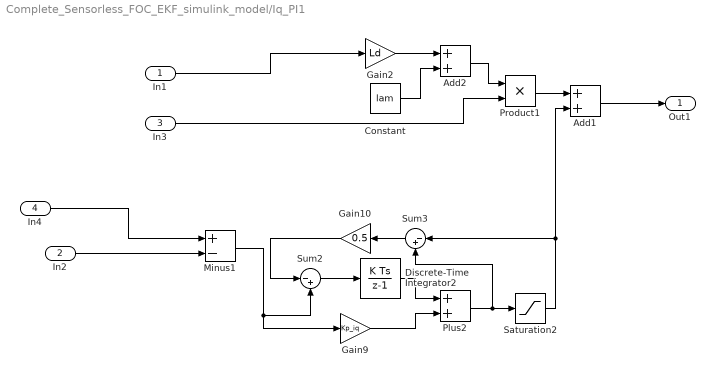
== system Complete_Sensorless_FOC_EKF_simulink_model/Iq_PI1 ==
  In1 : Inport
  In2 : Inport  Port=2
  In3 : Inport  Port=3
  In4 : Inport  Port=4
  Add1 : Sum
  Add2 : Sum
  Constant : Constant  Value=lam  VectorParams1D=off
  Discrete-Time Integrator2 : DiscreteIntegrator  gainval=Kp_iq  SampleTime=Ts  LimitOutput=on  UpperSaturationLimit=V_lim  LowerSaturationLimit=-V_lim  ICPrevOutput=DiscIntNeverNeededParam  ICPrevScaledInput=DiscIntNeverNeededParam
  Gain10 : Gain  Gain=0.5
  Gain2 : Gain  Gain=Ld
  Gain9 : Gain  Gain=Kp_iq
  Minus1 : Sum  Inputs=+-
  Plus2 : Sum
  Product1 : Product
  Saturation2 : Saturate  UpperLimit=V_lim  LowerLimit=-V_lim
  Sum2 : Sum  Inputs=|-+
  Sum3 : Sum  Inputs=|-+
  Out1 : Outport
  wires:
  Minus1/1 -> Sum2/2, Gain9/1
  Saturation2/1 -> Sum3/1, Add1/2
  Add2/1 -> Product1/1
  Gain2/1 -> Add2/1
  Constant/1 -> Add2/2
  In3/1 -> Product1/2
  Gain9/1 -> Plus2/2
  Discrete-Time Integrator2/1 -> Plus2/1
  Plus2/1 -> Sum3/2, Saturation2/1
  Gain10/1 -> Sum2/1
  In1/1 -> Gain2/1
  Sum2/1 -> Discrete-Time Integrator2/1
  Product1/1 -> Add1/1
  Sum3/1 -> Gain10/1
  Add1/1 -> Out1/1
  In2/1 -> Minus1/2
  In4/1 -> Minus1/1

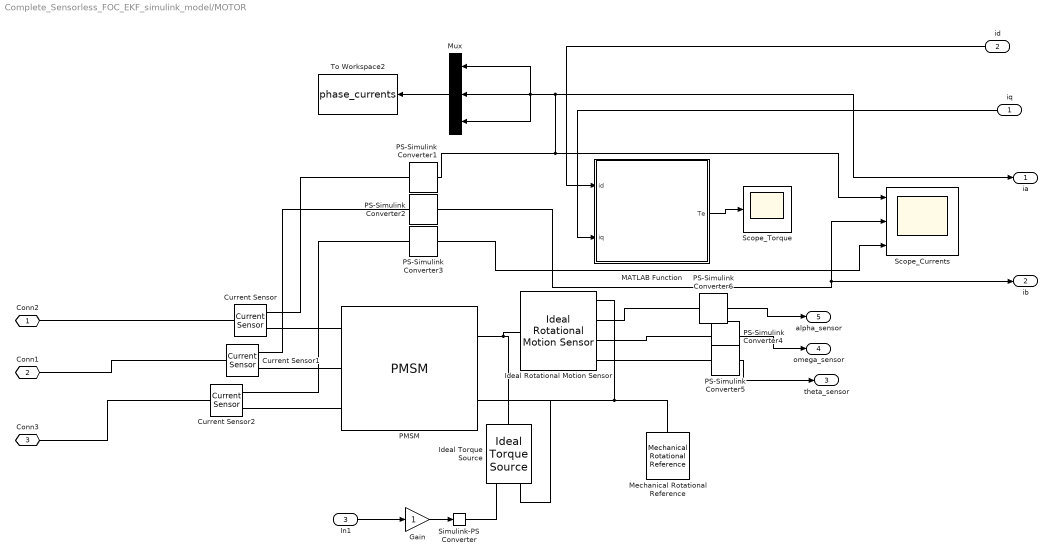
== system Complete_Sensorless_FOC_EKF_simulink_model/MOTOR ==
  iq : Inport
  id : Inport  Port=2
  In1 : Inport  Port=3
  Current Sensor : fl_lib/Electrical/Electrical Sensors/Current Sensor
  Current Sensor1 : fl_lib/Electrical/Electrical Sensors/Current Sensor
  Current Sensor2 : fl_lib/Electrical/Electrical Sensors/Current Sensor
  Gain : Gain
  Ideal Rotational Motion Sensor : fl_lib/Mechanical/Mechanical Sensors/Ideal Rotational Motion Sensor  reference=foundation.enum.MeasurementReference.difference  acceleration_port=true  velocity_port=true  position_port=true  wrap_angle=true  offset=0 rad
  Ideal Torque Source : fl_lib/Mechanical/Mechanical Sources/Ideal Torque Source
  MATLAB Function : MATLAB Function  TreatAsAtomicUnit=on
  Mechanical Rotational Reference : fl_lib/Mechanical/Rotational Elements/Mechanical Rotational Reference
  Mux : Mux  Inputs=3
  PMSM : ee_lib/Electromechanical/Permanent Magnet/PMSM  port_option=ee.enum.threePhasePort.expanded  winding_type=ee.enum.electromech.statorconfiguration.wye  machine_param=ee.enum.pmsm.parameterization.constant  nPolePairs=P  pmflux_param=ee.enum.pmflux.fluxlinkage  pm_flux_linkage=lam Wb  torque_constant=0.18 N*m/A  back_emf_constant=0.18 V*s/rad  stator_param=ee.enum.statorparam.LdLqL0  Ld=Ld H  Lq=Lq H  idVec=[-200, 0, 200] A  iqVec=[-200, 0, 200] A  LdMatrix=0.0002 * ones(3, 3) H  LqMatrix=0.0002 * ones(3, 3) H  PmMatrix=0.1 * ones(3, 3) Wb  ktMatrix=0.18 * ones(3, 3) N*m/A  keMatrix=0.18 * ones(3, 3) V*s/rad  L0=0.0085 H  Ls=0.0002 H  Lm=-0.00002 H  Ms=0.00002 H  Rs=Rs Ohm  zero_sequence=ee.enum.park.zerosequence.exclude  axes_param=ee.enum.rotorangle.daxis  loss_param=ee.enum.ironloss.none  losses_oc=[0, 0, 0] W  losses_sc=[0, 0, 0] W  f_losses=60 Hz  Isc_losses=95 A  J=J kg*m^2  lam=0.001 N*m*s/rad  i_d_specify=off  i_d_priority=None  i_d=0 A  i_d_nominal_specify=off  i_d_nominal_value=1  i_d_nominal_unit=A  i_q_specify=off  i_q_priority=None  i_q=0 A  i_q_nominal_specify=off  i_q_nominal_value=1  i_q_nominal_unit=A  torque_specify=off  torque_priority=None  torque=0 N*m  torque_nominal_specify=off  torque_nominal_value=1  torque_nominal_unit=N*m  angular_velocity_specify=on  angular_velocity_priority=High  angular_velocity=0 rad/s  angular_velocity_nominal_specify=off  angular_velocity_nominal_value=1  angular_velocity_nominal_unit=rpm  angular_position_specify=on  angular_position_priority=High  angular_position=pi/2 rad  angular_position_nominal_specify=off  angular_position_nominal_value=1  angular_position_nominal_unit=deg  alpha=3.93e-3 1/K  alpha_flux=-0.001 1/K  Tmeas=298.15 K  stator_thermal_mass=100 J/K  rotor_thermal_mass=200 J/K  Rm_percent_rotor=90  Rd_percent_rotor=30  temperatureA_specify=off  temperatureA_priority=High  temperatureA=25 degC  temperatureA_nominal_specify=off  temperatureA_nominal_value=1  temperatureA_nominal_unit=degC  temperatureB_specify=off  temperatureB_priority=High  temperatureB=25 degC  temperatureB_nominal_specify=off  temperatureB_nominal_value=1  temperatureB_nominal_unit=degC  temperatureC_specify=off  temperatureC_priority=High  temperatureC=25 degC  temperatureC_nominal_specify=off  temperatureC_nominal_value=1  temperatureC_nominal_unit=degC  temperatureR_specify=off  temperatureR_priority=High  temperatureR=25 degC  temperatureR_nominal_specify=off  temperatureR_nominal_value=1  temperatureR_nominal_unit=degC
  PS-Simulink Converter{1..6} (6 alike) : nesl_utility/PS-Simulink Converter  PhysicalDomain=network_engine_domain  SubClassName=ps_output  LeftPortType=input  RightPortType=output  PseudoPeriodic=off  Frequencies=[]  VectorFormat=inherit  Unit=inherit  AffineConversion=off
  Scope_Currents : Scope  NumInputPorts=3
      settings: ActiveDisplayYMinimum=-8.2949703721219432  ActiveDisplayYMaximum=9.3821609096223586  DataLoggingVariableName=currentData
  Scope_Torque : Scope
      settings: ActiveDisplayYMinimum=-2.01642745496106  ActiveDisplayYMaximum=3.2812220114633139  DataLoggingVariableName=ScopeData7
  Simulink-PS Converter : nesl_utility/Simulink-PS Converter  PhysicalDomain=network_engine_domain  SubClassName=ps_input  LeftPortType=input  RightPortType=output  PseudoPeriodic=off  Frequencies=[]  NoiseDistribution=none  NoiseParameters=[]  Unit=1  AffineConversion=off  FilteringAndDerivatives=zero  SimscapeFilterOrder=1  InputFilterTimeConstant=0.001  UdotUserProvided=0
  To Workspace2 : ToWorkspace  VariableName=phase_currents  SampleTime=-1
  Conn2 : PMIOPort  Side=Left
  Conn1 : PMIOPort  Port=2  Side=Left
  Conn3 : PMIOPort  Port=3  Side=Left
  ia : Outport
  ib : Outport  Port=2
  theta_sensor : Outport  Port=3
  omega_sensor : Outport  Port=4
  alpha_sensor : Outport  Port=5
  wires:
  PS-Simulink Converter1/1 -> Scope_Currents/1, ia/1, Mux/3, Mux/2, Mux/1
  PS-Simulink Converter4/1 -> omega_sensor/1
  MATLAB Function/1(Te) -> Scope_Torque/1
  iq/1 -> MATLAB Function/2(iq)
  PS-Simulink Converter2/1 -> Scope_Currents/2, ib/1
  PS-Simulink Converter3/1 -> Scope_Currents/3
  Mux/1 -> To Workspace2/1
  PS-Simulink Converter5/1 -> theta_sensor/1
  id/1 -> MATLAB Function/1(id)
  PS-Simulink Converter6/1 -> alpha_sensor/1
  In1/1 -> Gain/1
  Gain/1 -> Simulink-PS Converter/1
  connections:
  Current Sensor2/RConn1 -- PS-Simulink Converter3/LConn1
  Current Sensor1/RConn1 -- PS-Simulink Converter2/LConn1
  Current Sensor2/LConn1 -- Conn3/RConn1
  Ideal Rotational Motion Sensor/RConn1 -- Ideal Torque Source/RConn2 -- PMSM/RConn2 -- Mechanical Rotational Reference/LConn1
  Current Sensor2/RConn2 -- PMSM/LConn3
  Current Sensor/RConn2 -- PMSM/LConn1
  PS-Simulink Converter4/LConn1 -- Ideal Rotational Motion Sensor/RConn3
  Current Sensor/RConn1 -- PS-Simulink Converter1/LConn1
  Ideal Rotational Motion Sensor/LConn1 -- PMSM/RConn1 -- Ideal Torque Source/LConn1
  Ideal Rotational Motion Sensor/RConn4 -- PS-Simulink Converter5/LConn1
  PMSM/LConn2 -- Current Sensor1/RConn2
  Current Sensor1/LConn1 -- Conn1/RConn1
  Current Sensor/LConn1 -- Conn2/RConn1
  Ideal Rotational Motion Sensor/RConn2 -- PS-Simulink Converter6/LConn1
  Simulink-PS Converter/RConn1 -- Ideal Torque Source/RConn1

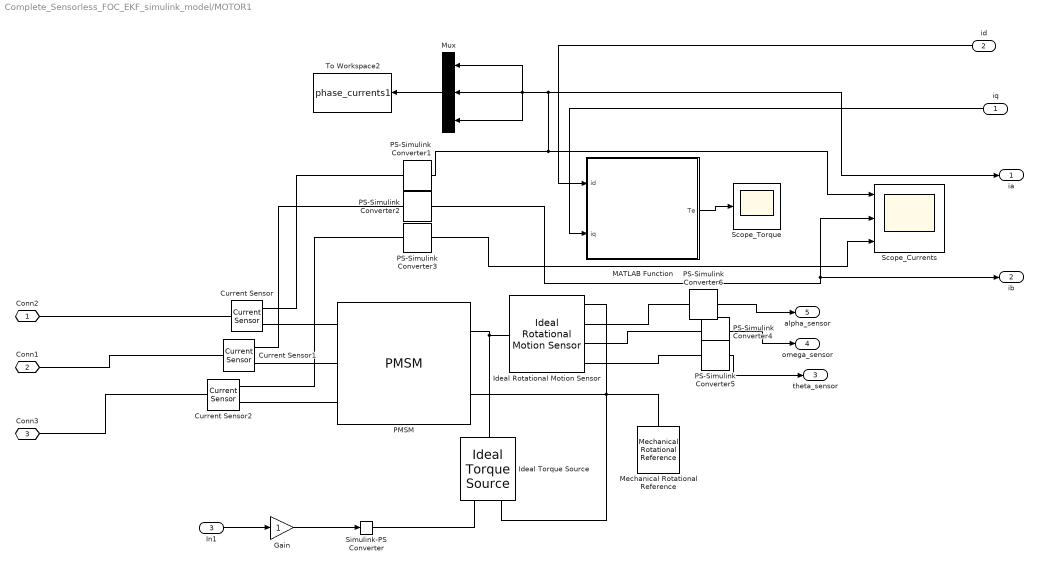
== system Complete_Sensorless_FOC_EKF_simulink_model/MOTOR1 ==
  iq : Inport
  id : Inport  Port=2
  In1 : Inport  Port=3
  Current Sensor : fl_lib/Electrical/Electrical Sensors/Current Sensor
  Current Sensor1 : fl_lib/Electrical/Electrical Sensors/Current Sensor
  Current Sensor2 : fl_lib/Electrical/Electrical Sensors/Current Sensor
  Gain : Gain
  Ideal Rotational Motion Sensor : fl_lib/Mechanical/Mechanical Sensors/Ideal Rotational Motion Sensor  reference=foundation.enum.MeasurementReference.difference  acceleration_port=true  velocity_port=true  position_port=true  wrap_angle=true  offset=0 rad
  Ideal Torque Source : fl_lib/Mechanical/Mechanical Sources/Ideal Torque Source
  MATLAB Function : MATLAB Function  TreatAsAtomicUnit=on
  Mechanical Rotational Reference : fl_lib/Mechanical/Rotational Elements/Mechanical Rotational Reference
  Mux : Mux  Inputs=3
  PMSM : ee_lib/Electromechanical/Permanent Magnet/PMSM  port_option=ee.enum.threePhasePort.expanded  winding_type=ee.enum.electromech.statorconfiguration.wye  machine_param=ee.enum.pmsm.parameterization.constant  nPolePairs=P  pmflux_param=ee.enum.pmflux.fluxlinkage  pm_flux_linkage=lam Wb  torque_constant=0.18 N*m/A  back_emf_constant=0.18 V*s/rad  stator_param=ee.enum.statorparam.LdLqL0  Ld=Ld H  Lq=Lq H  idVec=[-200, 0, 200] A  iqVec=[-200, 0, 200] A  LdMatrix=0.0002 * ones(3, 3) H  LqMatrix=0.0002 * ones(3, 3) H  PmMatrix=0.1 * ones(3, 3) Wb  ktMatrix=0.18 * ones(3, 3) N*m/A  keMatrix=0.18 * ones(3, 3) V*s/rad  L0=0.0085 H  Ls=0.0002 H  Lm=-0.00002 H  Ms=0.00002 H  Rs=Rs Ohm  zero_sequence=ee.enum.park.zerosequence.exclude  axes_param=ee.enum.rotorangle.daxis  loss_param=ee.enum.ironloss.none  losses_oc=[0, 0, 0] W  losses_sc=[0, 0, 0] W  f_losses=60 Hz  Isc_losses=95 A  J=J kg*m^2  lam=0.001 N*m*s/rad  i_d_specify=off  i_d_priority=None  i_d=0 A  i_d_nominal_specify=off  i_d_nominal_value=1  i_d_nominal_unit=A  i_q_specify=off  i_q_priority=None  i_q=0 A  i_q_nominal_specify=off  i_q_nominal_value=1  i_q_nominal_unit=A  torque_specify=off  torque_priority=None  torque=0 N*m  torque_nominal_specify=off  torque_nominal_value=1  torque_nominal_unit=N*m  angular_velocity_specify=on  angular_velocity_priority=High  angular_velocity=0 rad/s  angular_velocity_nominal_specify=off  angular_velocity_nominal_value=1  angular_velocity_nominal_unit=rpm  angular_position_specify=on  angular_position_priority=High  angular_position=pi/2 rad  angular_position_nominal_specify=off  angular_position_nominal_value=1  angular_position_nominal_unit=deg  alpha=3.93e-3 1/K  alpha_flux=-0.001 1/K  Tmeas=298.15 K  stator_thermal_mass=100 J/K  rotor_thermal_mass=200 J/K  Rm_percent_rotor=90  Rd_percent_rotor=30  temperatureA_specify=off  temperatureA_priority=High  temperatureA=25 degC  temperatureA_nominal_specify=off  temperatureA_nominal_value=1  temperatureA_nominal_unit=degC  temperatureB_specify=off  temperatureB_priority=High  temperatureB=25 degC  temperatureB_nominal_specify=off  temperatureB_nominal_value=1  temperatureB_nominal_unit=degC  temperatureC_specify=off  temperatureC_priority=High  temperatureC=25 degC  temperatureC_nominal_specify=off  temperatureC_nominal_value=1  temperatureC_nominal_unit=degC  temperatureR_specify=off  temperatureR_priority=High  temperatureR=25 degC  temperatureR_nominal_specify=off  temperatureR_nominal_value=1  temperatureR_nominal_unit=degC
  PS-Simulink Converter{1..6} (6 alike) : nesl_utility/PS-Simulink Converter  PhysicalDomain=network_engine_domain  SubClassName=ps_output  LeftPortType=input  RightPortType=output  PseudoPeriodic=off  Frequencies=[]  VectorFormat=inherit  Unit=inherit  AffineConversion=off
  Scope_Currents : Scope  NumInputPorts=3
      settings: ActiveDisplayYMinimum=-0.44861899872682687  ActiveDisplayYMaximum=0.54920756887767075  DataLoggingVariableName=currentData1
  Scope_Torque : Scope
      settings: ActiveDisplayYMinimum=-0.37165997601651568  ActiveDisplayYMaximum=1.6310198844793689  DataLoggingVariableName=ScopeData7
  Simulink-PS Converter : nesl_utility/Simulink-PS Converter  PhysicalDomain=network_engine_domain  SubClassName=ps_input  LeftPortType=input  RightPortType=output  PseudoPeriodic=off  Frequencies=[]  NoiseDistribution=none  NoiseParameters=[]  Unit=1  AffineConversion=off  FilteringAndDerivatives=zero  SimscapeFilterOrder=1  InputFilterTimeConstant=0.001  UdotUserProvided=0
  To Workspace2 : ToWorkspace  VariableName=phase_currents1  SampleTime=-1
  Conn2 : PMIOPort  Side=Left
  Conn1 : PMIOPort  Port=2  Side=Left
  Conn3 : PMIOPort  Port=3  Side=Left
  ia : Outport
  ib : Outport  Port=2
  theta_sensor : Outport  Port=3
  omega_sensor : Outport  Port=4
  alpha_sensor : Outport  Port=5
  wires:
  PS-Simulink Converter1/1 -> Scope_Currents/1, ia/1, Mux/3, Mux/2, Mux/1
  PS-Simulink Converter4/1 -> omega_sensor/1
  MATLAB Function/1(Te) -> Scope_Torque/1
  iq/1 -> MATLAB Function/2(iq)
  PS-Simulink Converter2/1 -> Scope_Currents/2, ib/1
  PS-Simulink Converter3/1 -> Scope_Currents/3
  Mux/1 -> To Workspace2/1
  PS-Simulink Converter5/1 -> theta_sensor/1
  id/1 -> MATLAB Function/1(id)
  PS-Simulink Converter6/1 -> alpha_sensor/1
  In1/1 -> Gain/1
  Gain/1 -> Simulink-PS Converter/1
  connections:
  Current Sensor2/RConn1 -- PS-Simulink Converter3/LConn1
  Current Sensor1/RConn1 -- PS-Simulink Converter2/LConn1
  Current Sensor2/LConn1 -- Conn3/RConn1
  Ideal Rotational Motion Sensor/RConn1 -- Ideal Torque Source/RConn2 -- PMSM/RConn2 -- Mechanical Rotational Reference/LConn1
  Current Sensor2/RConn2 -- PMSM/LConn3
  Current Sensor/RConn2 -- PMSM/LConn1
  PS-Simulink Converter4/LConn1 -- Ideal Rotational Motion Sensor/RConn3
  Current Sensor/RConn1 -- PS-Simulink Converter1/LConn1
  Ideal Rotational Motion Sensor/LConn1 -- PMSM/RConn1 -- Ideal Torque Source/LConn1
  Ideal Rotational Motion Sensor/RConn4 -- PS-Simulink Converter5/LConn1
  PMSM/LConn2 -- Current Sensor1/RConn2
  Current Sensor1/LConn1 -- Conn1/RConn1
  Current Sensor/LConn1 -- Conn2/RConn1
  Ideal Rotational Motion Sensor/RConn2 -- PS-Simulink Converter6/LConn1
  Simulink-PS Converter/RConn1 -- Ideal Torque Source/RConn1
